simulink model "Wind_Turbine"  (R2023a)
settings: Solver=ode1be  StartTime=0.0  StopTime=140  MaxStep=0.01  RelTol=1e-4  AbsTol=1e-4  EnableMultiTasking=on
PreLoadFcn:
  | warning off Simulink:Commands:LoadMdlParameterizedLink
PostLoadFcn:
  | warning off Simulink:blocks:MatchingGotoNotFound
  | warning off Simulink:blocks:MatchingFromNotFound
  | warning('off','Simulink:SL_OutputNotConnected');
  | warning off Simulink:Engine:SaveWithParameterizedLinks_Warning
  | warning off Simulink:Engine:SaveWithDisabledLinks_Warning
  | warning('off','Simulink:fixpoint:fxpParameterPrecisionLoss');
  | warning off Simulink:blocks:DTConversionUncessary
  | warning off ne_sli:simulator:input:FilteredInputs
  | warning off MATLAB:nearlySingularMatrix
  | 
  | warning off xPCTarget:modeloptions:StackIncrease
  | warning off xPCTarget:sampleTime:sampleTimeInvariance
  | warning off Simulink:blocks:TDelayFixedBuffer
  | 
  | Setup_WT_Configurations
StartFcn:
  | tic
StopFcn:
  | Elapsed_Sim_Time = toc;
  | disp(['Elapsed time is ' num2str(Elapsed_Sim_Time)]);
undefined symbols (not defined in the file or in its folder): radps2rpm, sigbuilder_block, WT_Params, X, Y, Z
libraries: sm_lib x6, Wind_Lib x4, fl_lib x4, Yaw_System_Lib x4, Geartrain_Lib x3, sdl_lib x3, Generator_Lib x3, Pitch_System_Lib x3, Pitch_Controller_Lib x3, Main_Controller_Lib x2, Hub_Axis_Lib x2, Blades_Lib x1
(part 2 of 2)

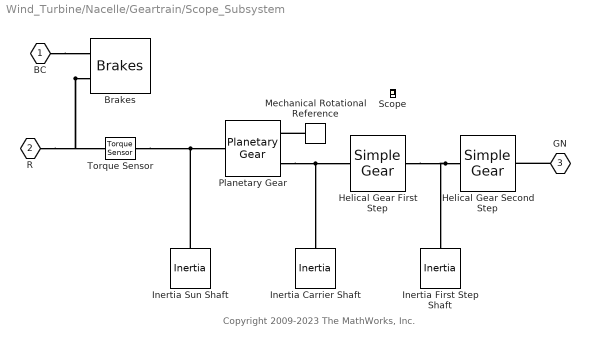
== system Wind_Turbine/Nacelle/Geartrain/Scope_Subsystem ==
  note: Copyright 2009-2023 The MathWorks, Inc.
  Brakes : Brakes_Lib/Brakes  SystemSampleTime=-1  VariantActivationTime=update diagram  Latency=0  AutoFrameSizeCalculation=off
  Helical Gear First Step : sdl_lib/Gears/Simple Gear  ratio=WT_Params.Geartrain.Gear_Ratio.first_step  rotation_direction=3-2*(2)  friction_model=1  T_noload=0.1 N*m  T_nom=5 N*m  efficiency_nom=0.8  efficiency=0.8  temperature_TLU=[ 280 300 320 ] K  load_TLU=[ 1 5 10 ] N*m  efficiency_TLU=[ 0.95 0.9 0.85 ]  efficiency_TLU2=[ 0.85 0.8 0.75; 0.95 0.9 0.85; 0.85 0.8 0.7 ]  w_thr=0.01 rad/s  pwr_thr=0.001 W  enable_backlash=false  hardstop_model=simscape.enum.hardstop.smooth  backlash_distance=1e-3 mm  r_base=0.1 m  transition=1e-4 mm  backlash_stiffness=1e7 N/m  backlash_damping=1e6 N*s/m  coeff_rest=0  v_tol=0.001 m/s  f_tol=0 N  mu_visc=[ 0 0 ] N*m/(rad/s)  enable_faults=simscape.enum.onoff.off  efficiency_fault=0.05  external_fault=simscape.enum.onoff.off  temporal_fault=simscape.enum.onoff.off  fault_time=5 s  fault_angles=pi / 12 rad  report_fault=(1)-1  thermal_mass=50 J/K  temperature_specify=off  temperature_priority=High  temperature=300 K  temperature_nominal_specify=off  temperature_nominal_unit=K  temperature_nominal_value=1  x_backlash_specify=off  x_backlash_priority=None  x_backlash=0 mm  x_backlash_nominal_specify=off  x_backlash_nominal_unit=mm  x_backlash_nominal_value=1  f_hardstop_specify=off  f_hardstop_priority=None  f_hardstop=0 N  f_hardstop_nominal_specify=off  f_hardstop_nominal_unit=N  f_hardstop_nominal_value=1  v_backlash_specify=off  v_backlash_priority=None  v_backlash=0 m/s  v_backlash_nominal_specify=off  v_backlash_nominal_unit=m/s  v_backlash_nominal_value=1
  Helical Gear Second Step : sdl_lib/Gears/Simple Gear  ratio=WT_Params.Geartrain.Gear_Ratio.second_step_primary_generator  rotation_direction=3-2*(2)  friction_model=1  T_noload=0.1 N*m  T_nom=5 N*m  efficiency_nom=0.8  efficiency=0.8  temperature_TLU=[ 280 300 320 ] K  load_TLU=[ 1 5 10 ] N*m  efficiency_TLU=[ 0.95 0.9 0.85 ]  efficiency_TLU2=[ 0.85 0.8 0.75; 0.95 0.9 0.85; 0.85 0.8 0.7 ]  w_thr=0.01 rad/s  pwr_thr=0.001 W  enable_backlash=false  hardstop_model=simscape.enum.hardstop.smooth  backlash_distance=1e-3 mm  r_base=0.1 m  transition=1e-4 mm  backlash_stiffness=1e7 N/m  backlash_damping=1e6 N*s/m  coeff_rest=0  v_tol=0.001 m/s  f_tol=0 N  mu_visc=[ 0 0 ] N*m/(rad/s)  enable_faults=simscape.enum.onoff.off  efficiency_fault=0.05  external_fault=simscape.enum.onoff.off  temporal_fault=simscape.enum.onoff.off  fault_time=5 s  fault_angles=pi / 12 rad  report_fault=(1)-1  thermal_mass=50 J/K  temperature_specify=off  temperature_priority=High  temperature=300 K  temperature_nominal_specify=off  temperature_nominal_unit=K  temperature_nominal_value=1  x_backlash_specify=off  x_backlash_priority=None  x_backlash=0 mm  x_backlash_nominal_specify=off  x_backlash_nominal_unit=mm  x_backlash_nominal_value=1  f_hardstop_specify=off  f_hardstop_priority=None  f_hardstop=0 N  f_hardstop_nominal_specify=off  f_hardstop_nominal_unit=N  f_hardstop_nominal_value=1  v_backlash_specify=off  v_backlash_priority=None  v_backlash=0 m/s  v_backlash_nominal_specify=off  v_backlash_nominal_unit=m/s  v_backlash_nominal_value=1
  Inertia Carrier Shaft : fl_lib/Mechanical/Rotational Elements/Inertia  inertia=WT_Params.Geartrain.inertia_sun_shaft kg*m^2  num_ports=foundation.enum.numPorts2.one  w_specify=on  w_priority=High  w=0 rad/s  w_nominal_specify=off  w_nominal_unit=rad/s  w_nominal_value=1  t_specify=off  t_priority=High  t=0 N*m  t_nominal_specify=off  t_nominal_unit=N*m  t_nominal_value=1
  Inertia First Step Shaft : fl_lib/Mechanical/Rotational Elements/Inertia  inertia=WT_Params.Geartrain.inertia_first_step_shaft kg*m^2  num_ports=foundation.enum.numPorts2.one  w_specify=on  w_priority=High  w=0 rad/s  w_nominal_specify=off  w_nominal_unit=rad/s  w_nominal_value=1  t_specify=off  t_priority=High  t=0 N*m  t_nominal_specify=off  t_nominal_unit=N*m  t_nominal_value=1
  Inertia Sun Shaft : fl_lib/Mechanical/Rotational Elements/Inertia  inertia=WT_Params.Geartrain.inertia_sun_shaft kg*m^2  num_ports=foundation.enum.numPorts2.one  w_specify=on  w_priority=High  w=0 rad/s  w_nominal_specify=off  w_nominal_unit=rad/s  w_nominal_value=1  t_specify=off  t_priority=High  t=0 N*m  t_nominal_specify=off  t_nominal_unit=N*m  t_nominal_value=1
  Mechanical Rotational Reference : fl_lib/Mechanical/Rotational Elements/Mechanical Rotational Reference
  Planetary Gear : sdl_lib/Gears/Planetary Gear  rs_ratio=WT_Params.Geartrain.Gear_Ratio.planetary  friction_model=sdl.enum.gear_friction.constant  efficiency=[ 0.7 0.7 ]  temperature_TLU=[ 280 300 320 ] K  efficiency_sp_TLU=[ 0.95 0.9 0.85 ]  efficiency_rp_TLU=[ 0.95 0.9 0.85 ]  pwr_thr=[ 0.001 0.001 ] W  mu_visc=WT_Params.Geartrain.Planetary.viscous_losses N*m/(rad/s)  model_inertia=0  planet_inertia=0.001 kg*m^2  thermal_mass=50 J/K  T_init=300 K
  Scope : Scope
  Torque Sensor : Geartrain_Lib/Ideal/Torque Sensor  SystemSampleTime=-1  VariantActivationTime=update diagram  Latency=0  AutoFrameSizeCalculation=off
  BC : PMIOPort  Side=Left
  R : PMIOPort  Port=2  Side=Left
  GN : PMIOPort  Port=3  Side=Right
  connections:
  Helical Gear Second Step/RConn1 -- Inertia First Step Shaft/LConn1 -- Helical Gear First Step/LConn1
  Planetary Gear/RConn2 -- Inertia Carrier Shaft/LConn1 -- Helical Gear First Step/RConn1
  Inertia Sun Shaft/LConn1 -- Torque Sensor/RConn1 -- Planetary Gear/LConn1
  Brakes/LConn2 -- R/RConn1 -- Torque Sensor/LConn1
  GN/RConn1 -- Helical Gear Second Step/LConn1
  BC/RConn1 -- Brakes/LConn1
  Mechanical Rotational Reference/LConn1 -- Planetary Gear/RConn1

== system Wind_Turbine/Scopes/Configure Turbine/Subsystem ==

== system Wind_Turbine/Scopes/Configure Turbine/Subsystem1 ==

== system Wind_Turbine/Scopes/Configure Turbine/Subsystem10 ==

== system Wind_Turbine/Scopes/Configure Turbine/Subsystem11 ==

== system Wind_Turbine/Scopes/Configure Turbine/Subsystem12 ==

== system Wind_Turbine/Scopes/Configure Turbine/Subsystem13 ==

== system Wind_Turbine/Scopes/Configure Turbine/Subsystem14 ==

== system Wind_Turbine/Scopes/Configure Turbine/Subsystem15 ==

== system Wind_Turbine/Scopes/Configure Turbine/Subsystem16 ==

== system Wind_Turbine/Scopes/Configure Turbine/Subsystem17 ==

== system Wind_Turbine/Scopes/Configure Turbine/Subsystem18 ==

== system Wind_Turbine/Scopes/Configure Turbine/Subsystem19 ==

== system Wind_Turbine/Scopes/Configure Turbine/Subsystem2 ==

== system Wind_Turbine/Scopes/Configure Turbine/Subsystem20 ==

== system Wind_Turbine/Scopes/Configure Turbine/Subsystem21 ==

== system Wind_Turbine/Scopes/Configure Turbine/Subsystem22 ==

== system Wind_Turbine/Scopes/Configure Turbine/Subsystem23 ==

== system Wind_Turbine/Scopes/Configure Turbine/Subsystem24 ==

== system Wind_Turbine/Scopes/Configure Turbine/Subsystem3 ==

== system Wind_Turbine/Scopes/Configure Turbine/Subsystem4 ==

== system Wind_Turbine/Scopes/Configure Turbine/Subsystem5 ==

== system Wind_Turbine/Scopes/Configure Turbine/Subsystem6 ==

== system Wind_Turbine/Scopes/Configure Turbine/Subsystem7 ==

== system Wind_Turbine/Scopes/Configure Turbine/Subsystem8 ==

== system Wind_Turbine/Scopes/Configure Turbine/Subsystem9 ==

== system Wind_Turbine/Turbine Input/Commands/Signal Builder ==
  Demux : Demux  Tag=STV Demux  Outputs=1
      settings: DisplayOption=none
  FromWs : FromWorkspace  Tag=STV FromWs  VariableName=tuvar
      SigBuilderData=|
      | common.afterFinalStr = 'Extrapolate'
      | common.sampleTime = 0
      | dataSet(1).timeRange = [0 50]
      | dataSet(1).name = 'Pos_Test'
      | dataSet(2).timeRange = [0 50]
      | dataSet(2).name = 'Pos_Neg_Test'
      | dataSet(3).timeRange = [0 50]
      | dataSet(3).name = 'Step_Test'
      | sbobj.Groups(1).Name = 'Pos_Test'
      | sbobj.Groups(1).Signals.Name = 'Signal 1'
      | sbobj.Groups(1).Signals.XData = [0 5 5 7.5 7.5 25.1 25.1 28 28 50]
      | sbobj.Groups(1).Signals.YData = [0 0 20 20 0 0 20 20 0 0]
      | sbobj.Groups(1).TimeRange = [0 50]
      | sbobj.Groups(2).Name = 'Pos_Neg_Test'
      | sbobj.Groups(2).Signals.Name = 'Signal 1'
      | sbobj.Groups(2).Signals.XData = [0 3 3 5.5 5.5 8 8 10.5 10.5 50]
      | sbobj.Groups(2).Signals.YData = [0 0 20 20 0 0 -20 -20 0 0]
      | sbobj.Groups(2).TimeRange = [0 50]
      | sbobj.Groups(3).Name = 'Step_Test'
      | sbobj.Groups(3).Signals.Name = 'Signal 1'
      | sbobj.Groups(3).Signals.XData = [0 1 1 7.5 25.1 30 30 50]
      | sbobj.Groups(3).Signals.YData = [0 0 20 20 20 20 0 0]
      | sbobj.Groups(3).TimeRange = [0 50]
  Signal 1 : Outport  Tag=STV Outport  VectorParamsAs1DForOutWhenUnconnected=off
  wires:
  Demux/1 -> Signal 1/1
  FromWs/1 -> Demux/1

== system Wind_Turbine/Turbine Input/Commands/Signal Builder2 ==
  Demux : Demux  Tag=STV Demux  Outputs=1
      settings: DisplayOption=none
  FromWs : FromWorkspace  Tag=STV FromWs  VariableName=tuvar
      SigBuilderData=|
      | common.afterFinalStr = 'Extrapolate'
      | common.sampleTime = 0
      | dataSet(1).timeRange = [0 50]
      | dataSet(1).name = 'Pos_Neg_Test'
      | dataSet(2).timeRange = [0 50]
      | dataSet(2).name = 'Step_Test'
      | dataSet(3).timeRange = [0 50]
      | dataSet(3).name = 'Ramp_Test'
      | sbobj.Groups(1).Name = 'Pos_Neg_Test'
      | sbobj.Groups(1).Signals.Name = 'Signal 1'
      | sbobj.Groups(1).Signals.XData = [0 1 1 11 11 21 21 31 31 50]
      | sbobj.Groups(1).Signals.YData = [0 0 4 4 0 0 -4 -4 0 0]
      | sbobj.Groups(2).Name = 'Step_Test'
      | sbobj.Groups(2).Signals.Name = 'Signal 1'
      | sbobj.Groups(2).Signals.XData = [0 1 1 11 21 31 31 50]
      | sbobj.Groups(2).Signals.YData = [0 0 4 4 4 4 0 0]
      | sbobj.Groups(3).Name = 'Ramp_Test'
      | sbobj.Groups(3).Signals.Name = 'Signal 1'
      | sbobj.Groups(3).Signals.XData = [0 1 1 11 21 31 39.1 50]
      | sbobj.Groups(3).Signals.YData = [0 0 2.46 4 2.32 3.18 1.16 0]
  Signal 1 : Outport  Tag=STV Outport  VectorParamsAs1DForOutWhenUnconnected=off
  wires:
  Demux/1 -> Signal 1/1
  FromWs/1 -> Demux/1

== system Wind_Turbine/Turbine Input/Wind/Wind Input ==
  Demux : Demux  Tag=STV Demux  Outputs=3
      settings: DisplayOption=none
  FromWs : FromWorkspace  Tag=STV FromWs  VariableName=tuvar
      SigBuilderData=|
      | common.afterFinalStr = 'Extrapolate'
      | common.sampleTime = 0
      | dataSet(1).timeRange = [0 130]
      | dataSet(1).name = 'Constant Wind No Yaw'
      | dataSet(2).timeRange = [0 130]
      | dataSet(2).name = 'Constant Wind'
      | dataSet(3).timeRange = [0 130]
      | dataSet(3).name = 'High Wind Speed'
      | dataSet(4).timeRange = [0 130]
      | dataSet(4).name = 'Cut Out'
      | dataSet(5).timeRange = [0 60]
      | dataSet(5).name = 'Start Stop'
      | dataSet(6).timeRange = [0 130]
      | dataSet(6).name = 'Start Stop No Yaw'
      | dataSet(7).timeRange = [0 130]
      | dataSet(7).name = 'Varying Wind'
      | sbobj.Groups(1).Name = 'Constant Wind No Yaw'
      | sbobj.Groups(1).Signals(1).Name = 'Wind Speed'
      | sbobj.Groups(1).Signals(1).XData = [0 10 130]
      | sbobj.Groups(1).Signals(1).YData = [10 10 10]
      | sbobj.Groups(1).Signals(2).Name = 'Wind Direction'
      | sbobj.Groups(1).Signals(2).XData = [0 1 11 21 31 130]
      | sbobj.Groups(1).Signals(2).YData = [0 0 0 0 0 0]
      | sbobj.Groups(1).Signals(3).Name = 'Signal 1'
      | sbobj.Groups(1).Signals(3).XData = [0 2.72727272727 5.45454545455 8.18181818182 10.9090909091 13.6363636364 16.3636363636 19.0909090909 21.8181818182 24.5454545455 27.2727272727 30 32.7272727273 35.4545454545 38.1818181818 40.9090909091 43.6363636364 46.3636363636 49.0909090909 51.8181818182 54.5454545455 57.2727272727 60 62.7272727273 65.4545454545 68.1818181818 70.9090909091 73.6363636364 76.3636363636 79.0909090909 81.8181818182 84.5454545455 87.2727272727 90 92.7272727273 95.4545454545 98.1818181818 100.909090909 103.636363636 106.363636364 109.090909091 111.818181818 114.545454545 117.272727273 120 122.727272727 125.454545455 128.181818182 130]
      | sbobj.Groups(1).Signals(3).YData = [12.5 13.8516020436 14.7740799884 14.9745536047 14.3893739359 13.2043313921 11.7956686079 10.6106260641 10.0254463953 10.2259200116 11.1483979564 12.5 13.8516020436 14.7740799884 14.9745536047 14.3893739359 13.2043313921 11.7956686079 10.6106260641 10.0254463953 10.2259200116 11.1483979564 12.5 13.8516020436 14.7740799884 14.9745536047 14.3893739359 13.2043313921 11.7956686079 10.6106260641 10.0254463953 10.2259200116 11.1483979564 12.5 13.8516020436 14.7740799884 14.9745536047 14.3893739359 13.2043313921 11.7956686079 10.6106260641 10.0254463953 10.2259200116 11.1483979564 12.5 13.8516020436 14.7740799884 14.9745536047 14.6650635095]
      | sbobj.Groups(1).TimeRange = [0 130]
      | sbobj.Groups(2).Name = 'Constant Wind'
      | sbobj.Groups(2).Signals(1).Name = 'Wind Speed'
      | sbobj.Groups(2).Signals(1).XData = [0 10 130]
      | sbobj.Groups(2).Signals(1).YData = [10 10 10]
      | sbobj.Groups(2).Signals(2).Name = 'Wind Direction'
      | sbobj.Groups(2).Signals(2).XData = [0 1 1 11 11 21 21 31 31 130]
      | sbobj.Groups(2).Signals(2).YData = [0 0 4 4 0 0 -4 -4 0 0]
      | sbobj.Groups(2).Signals(3).Name = 'Signal 1'
      | sbobj.Groups(2).Signals(3).XData = [0 2.72727272727 5.45454545455 8.18181818182 10.9090909091 13.6363636364 16.3636363636 19.0909090909 21.8181818182 24.5454545455 27.2727272727 30 32.7272727273 35.4545454545 38.1818181818 40.9090909091 43.6363636364 46.3636363636 49.0909090909 51.8181818182 54.5454545455 57.2727272727 60 62.7272727273 65.4545454545 68.1818181818 70.9090909091 73.6363636364 76.3636363636 79.0909090909 81.8181818182 84.5454545455 87.2727272727 90 92.7272727273 95.4545454545 98.1818181818 100.909090909 103.636363636 106.363636364 109.090909091 111.818181818 114.545454545 117.272727273 120 122.727272727 125.454545455 128.181818182 130]
      | sbobj.Groups(2).Signals(3).YData = [12.5 13.8516020436 14.7740799884 14.9745536047 14.3893739359 13.2043313921 11.7956686079 10.6106260641 10.0254463953 10.2259200116 11.1483979564 12.5 13.8516020436 14.7740799884 14.9745536047 14.3893739359 13.2043313921 11.7956686079 10.6106260641 10.0254463953 10.2259200116 11.1483979564 12.5 13.8516020436 14.7740799884 14.9745536047 14.3893739359 13.2043313921 11.7956686079 10.6106260641 10.0254463953 10.2259200116 11.1483979564 12.5 13.8516020436 14.7740799884 14.9745536047 14.3893739359 13.2043313921 11.7956686079 10.6106260641 10.0254463953 10.2259200116 11.1483979564 12.5 13.8516020436 14.7740799884 14.9745536047 14.6650635095]
      | sbobj.Groups(2).TimeRange = [0 130]
      | sbobj.Groups(3).Name = 'High Wind Speed'
      | sbobj.Groups(3).Signals(1).Name = 'Wind Speed'
      | sbobj.Groups(3).Signals(1).XData = [0 10 60 130]
      | sbobj.Groups(3).Signals(1).YData = [10 10 10 10]
      | sbobj.Groups(3).Signals(2).Name = 'Wind Direction'
      | sbobj.Groups(3).Signals(2).XData = [0 10 11 20 30 60 130]
      | sbobj.Groups(3).Signals(2).YData = [0 0.1 0.11 0.2 0.3 0.6 1.3]
      | sbobj.Groups(3).Signals(3).Name = 'Signal 1'
      | sbobj.Groups(3).Signals(3).XData = [0 2.72727272727 5.45454545455 8.18181818182 10.9090909091 13.6363636364 16.3636363636 19.0909090909 21.8181818182 24.5454545455 27.2727272727 30 32.7272727273 35.4545454545 38.1818181818 40.9090909091 43.6363636364 46.3636363636 49.0909090909 51.8181818182 54.5454545455 57.2727272727 60 62.7272727273 65.4545454545 68.1818181818 70.9090909091 73.6363636364 76.3636363636 79.0909090909 81.8181818182 84.5454545455 87.2727272727 90 92.7272727273 95.4545454545 98.1818181818 100.909090909 103.636363636 106.363636364 109.090909091 111.818181818 114.545454545 117.272727273 120 122.727272727 125.454545455 128.181818182 130]
      | sbobj.Groups(3).Signals(3).YData = [12.5 13.8516020436 14.7740799884 14.9745536047 14.3893739359 13.2043313921 11.7956686079 10.6106260641 10.0254463953 10.2259200116 11.1483979564 12.5 13.8516020436 14.7740799884 14.9745536047 14.3893739359 13.2043313921 11.7956686079 10.6106260641 10.0254463953 10.2259200116 11.1483979564 12.5 13.8516020436 14.7740799884 14.9745536047 14.3893739359 13.2043313921 11.7956686079 10.6106260641 10.0254463953 10.2259200116 11.1483979564 12.5 13.8516020436 14.7740799884 14.9745536047 14.3893739359 13.2043313921 11.7956686079 10.6106260641 10.0254463953 10.2259200116 11.1483979564 12.5 13.8516020436 14.7740799884 14.9745536047 14.6650635095]
      | sbobj.Groups(3).TimeRange = [0 130]
      | sbobj.Groups(4).Name = 'Cut Out'
      | sbobj.Groups(4).Signals(1).Name = 'Wind Speed'
      | sbobj.Groups(4).Signals(1).XData = [0 5 25.1 28 60 75 121.8 130]
      | sbobj.Groups(4).Signals(1).YData = [10 10 8.7 7.85 9.65 2 2 2]
      | sbobj.Groups(4).Signals(2).Name = 'Wind Direction'
      | sbobj.Groups(4).Signals(2).XData = [0 1 1 11 11 21 21 31 31 130]
      | sbobj.Groups(4).Signals(2).YData = [0 0 4 4 0 0 -4 -4 0 0]
      | sbobj.Groups(4).Signals(3).Name = 'Signal 1'
      | sbobj.Groups(4).Signals(3).XData = [0 2.72727272727 5.45454545455 8.18181818182 10.9090909091 13.6363636364 16.3636363636 19.0909090909 21.8181818182 24.5454545455 27.2727272727 30 32.7272727273 35.4545454545 38.1818181818 40.9090909091 43.6363636364 46.3636363636 49.0909090909 51.8181818182 54.5454545455 57.2727272727 60 62.7272727273 65.4545454545 68.1818181818 70.9090909091 73.6363636364 76.3636363636 79.0909090909 81.8181818182 84.5454545455 87.2727272727 90 92.7272727273 95.4545454545 98.1818181818 100.909090909 103.636363636 106.363636364 109.090909091 111.818181818 114.545454545 117.272727273 120 122.727272727 125.454545455 128.181818182 130]
      | sbobj.Groups(4).Signals(3).YData = [12.5 13.8516020436 14.7740799884 14.9745536047 14.3893739359 13.2043313921 11.7956686079 10.6106260641 10.0254463953 10.2259200116 11.1483979564 12.5 13.8516020436 14.7740799884 14.9745536047 14.3893739359 13.2043313921 11.7956686079 10.6106260641 10.0254463953 10.2259200116 11.1483979564 12.5 13.8516020436 14.7740799884 14.9745536047 14.3893739359 13.2043313921 11.7956686079 10.6106260641 10.0254463953 10.2259200116 11.1483979564 12.5 13.8516020436 14.7740799884 14.9745536047 14.3893739359 13.2043313921 11.7956686079 10.6106260641 10.0254463953 10.2259200116 11.1483979564 12.5 13.8516020436 14.7740799884 14.9745536047 14.6650635095]
      | sbobj.Groups(4).TimeRange = [0 130]
      | sbobj.Groups(5).Name = 'Start Stop'
      | sbobj.Groups(5).Signals(1).Name = 'Wind Speed'
      | sbobj.Groups(5).Signals(1).XData = [0 10 20 30 60 130]
      | sbobj.Groups(5).Signals(1).YData = [0 10 20 30 60 60]
      | sbobj.Groups(5).Signals(2).Name = 'Wind Direction'
      | sbobj.Groups(5).Signals(2).XData = [0 1 10 20 31 36.6 54.8 130]
      | sbobj.Groups(5).Signals(2).YData = [0 0 0 0 0 0 0 0]
      | sbobj.Groups(5).Signals(3).Name = 'Signal 1'
      | sbobj.Groups(5).Signals(3).XData = [0 2.72727272727 5.45454545455 8.18181818182 10.9090909091 13.6363636364 16.3636363636 19.0909090909 21.8181818182 24.5454545455 27.2727272727 30 32.7272727273 35.4545454545 38.1818181818 40.9090909091 43.6363636364 46.3636363636 49.0909090909 51.8181818182 54.5454545455 57.2727272727 60 62.7272727273 65.4545454545 68.1818181818 70.9090909091 73.6363636364 76.3636363636 79.0909090909 81.8181818182 84.5454545455 87.2727272727 90 92.7272727273 95.4545454545 98.1818181818 100.909090909 103.636363636 106.363636364 109.090909091 111.818181818 114.545454545 117.272727273 120 122.727272727 125.454545455 128.181818182 130]
      | sbobj.Groups(5).Signals(3).YData = [12.5 13.8516020436 14.7740799884 14.9745536047 14.3893739359 13.2043313921 11.7956686079 10.6106260641 10.0254463953 10.2259200116 11.1483979564 12.5 13.8516020436 14.7740799884 14.9745536047 14.3893739359 13.2043313921 11.7956686079 10.6106260641 10.0254463953 10.2259200116 11.1483979564 12.5 13.8516020436 14.7740799884 14.9745536047 14.3893739359 13.2043313921 11.7956686079 10.6106260641 10.0254463953 10.2259200116 11.1483979564 12.5 13.8516020436 14.7740799884 14.9745536047 14.3893739359 13.2043313921 11.7956686079 10.6106260641 10.0254463953 10.2259200116 11.1483979564 12.5 13.8516020436 14.7740799884 14.9745536047 14.6650635095]
      | sbobj.Groups(5).TimeRange = [0 130]
      | sbobj.Groups(6).Name = 'Start Stop No Yaw'
      | sbobj.Groups(6).Signals(1).Name = 'Wind Speed'
      | sbobj.Groups(6).Signals(1).XData = [0 5 25 28 55 75 80 130]
      | sbobj.Groups(6).Signals(1).YData = [2 2 13 10 15 2 2 2]
      | sbobj.Groups(6).Signals(2).Name = 'Wind Direction'
      | sbobj.Groups(6).Signals(2).XData = [0 130]
      | sbobj.Groups(6).Signals(2).YData = [0 0]
      | sbobj.Groups(6).Signals(3).Name = 'Signal 1'
      | sbobj.Groups(6).Signals(3).XData = [0 2.72727272727 5.45454545455 8.18181818182 10.9090909091 13.6363636364 16.3636363636 19.0909090909 21.8181818182 24.5454545455 27.2727272727 30 32.7272727273 35.4545454545 38.1818181818 40.9090909091 43.6363636364 46.3636363636 49.0909090909 51.8181818182 54.5454545455 57.2727272727 60 62.7272727273 65.4545454545 68.1818181818 70.9090909091 73.6363636364 76.3636363636 79.0909090909 81.8181818182 84.5454545455 87.2727272727 90 92.7272727273 95.4545454545 98.1818181818 100.909090909 103.636363636 106.363636364 109.090909091 111.818181818 114.545454545 117.272727273 120 122.727272727 125.454545455 128.181818182 130]
      | sbobj.Groups(6).Signals(3).YData = [12.5 13.8516020436 14.7740799884 14.9745536047 14.3893739359 13.2043313921 11.7956686079 10.6106260641 10.0254463953 10.2259200116 11.1483979564 12.5 13.8516020436 14.7740799884 14.9745536047 14.3893739359 13.2043313921 11.7956686079 10.6106260641 10.0254463953 10.2259200116 11.1483979564 12.5 13.8516020436 14.7740799884 14.9745536047 14.3893739359 13.2043313921 11.7956686079 10.6106260641 10.0254463953 10.2259200116 11.1483979564 12.5 13.8516020436 14.7740799884 14.9745536047 14.3893739359 13.2043313921 11.7956686079 10.6106260641 10.0254463953 10.2259200116 11.1483979564 12.5 13.8516020436 14.7740799884 14.9745536047 14.6650635095]
      | sbobj.Groups(6).TimeRange = [0 130]
      | sbobj.Groups(7).Name = 'Varying Wind'
      | sbobj.Groups(7).Signals(1).Name = 'Wind Speed'
      | sbobj.Groups(7).Signals(1).XData = [0 5 25 28 45 60.2 75 78.2 80 130]
      | sbobj.Groups(7).Signals(1).YData = [2 2 13 10 14.4 10.6 13.9 8 8 2]
      | sbobj.Groups(7).Signals(2).Name = 'Wind Direction'
      | sbobj.Groups(7).Signals(2).XData = [0 1 11 21 31 36.6 54.8 75 130]
      | sbobj.Groups(7).Signals(2).YData = [0 0 2.9 0.5 0.5 1.57171717172 -4 -4 -4]
      | sbobj.Groups(7).Signals(3).Name = 'Signal 1'
      | sbobj.Groups(7).Signals(3).XData = [0 2.72727272727 5.45454545455 8.18181818182 10.9090909091 13.6363636364 16.3636363636 19.0909090909 21.8181818182 24.5454545455 27.2727272727 30 32.7272727273 35.4545454545 38.1818181818 40.9090909091 43.6363636364 46.3636363636 49.0909090909 51.8181818182 54.5454545455 57.2727272727 60 62.7272727273 65.4545454545 68.1818181818 70.9090909091 73.6363636364 76.3636363636 79.0909090909 81.8181818182 84.5454545455 87.2727272727 90 92.7272727273 95.4545454545 98.1818181818 100.909090909 103.636363636 106.363636364 109.090909091 111.818181818 114.545454545 117.272727273 120 122.727272727 125.454545455 128.181818182 130]
      | sbobj.Groups(7).Signals(3).YData = [12.5 13.8516020436 14.7740799884 14.9745536047 14.3893739359 13.2043313921 11.7956686079 10.6106260641 10.0254463953 10.2259200116 11.1483979564 12.5 13.8516020436 14.7740799884 14.9745536047 14.3893739359 13.2043313921 11.7956686079 10.6106260641 10.0254463953 10.2259200116 11.1483979564 12.5 13.8516020436 14.7740799884 14.9745536047 14.3893739359 13.2043313921 11.7956686079 10.6106260641 10.0254463953 10.2259200116 11.1483979564 12.5 13.8516020436 14.7740799884 14.9745536047 14.3893739359 13.2043313921 11.7956686079 10.6106260641 10.0254463953 10.2259200116 11.1483979564 12.5 13.8516020436 14.7740799884 14.9745536047 14.6650635095]
      | sbobj.Groups(7).TimeRange = [0 130]
  Wind Speed : Outport  Tag=STV Outport  VectorParamsAs1DForOutWhenUnconnected=off
  Wind Direction : Outport  Tag=STV Outport  Port=2  VectorParamsAs1DForOutWhenUnconnected=off
  Signal 1 : Outport  Tag=STV Outport  Port=3
  wires:
  Demux/2 -> Wind Direction/1
  Demux/1 -> Wind Speed/1
  FromWs/1 -> Demux/1
  Demux/3 -> Signal 1/1
